simulink model "CanBusRagnarPacketLoss"  (R2021b)
settings: Solver=VariableStepAuto  StartTime=0.0  StopTime=6  RelTol=1e-3
values from neighbouring files (symbols this model uses):
  sys_mimo = ss(A,B,C,0)    [SS_MIMO.m]
libraries: truetime x6, simulink_extras x2, dspsrcs4 x1
settings Model: Creator=mozzr  LastModifiedBy=mozzr
settings SolverCC: AlgebraicLoopSolver=TrustRegion

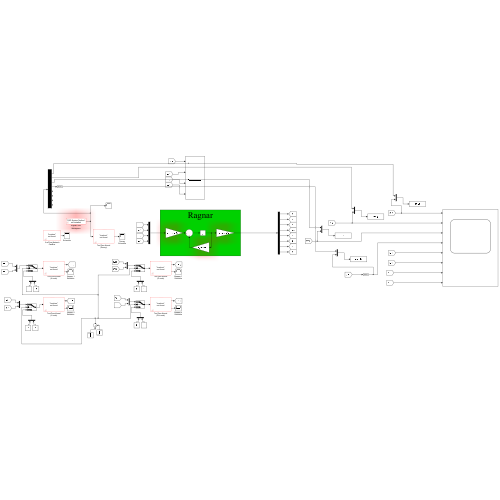
[thumbnail: Simulink's stored preview of the top-level diagram]
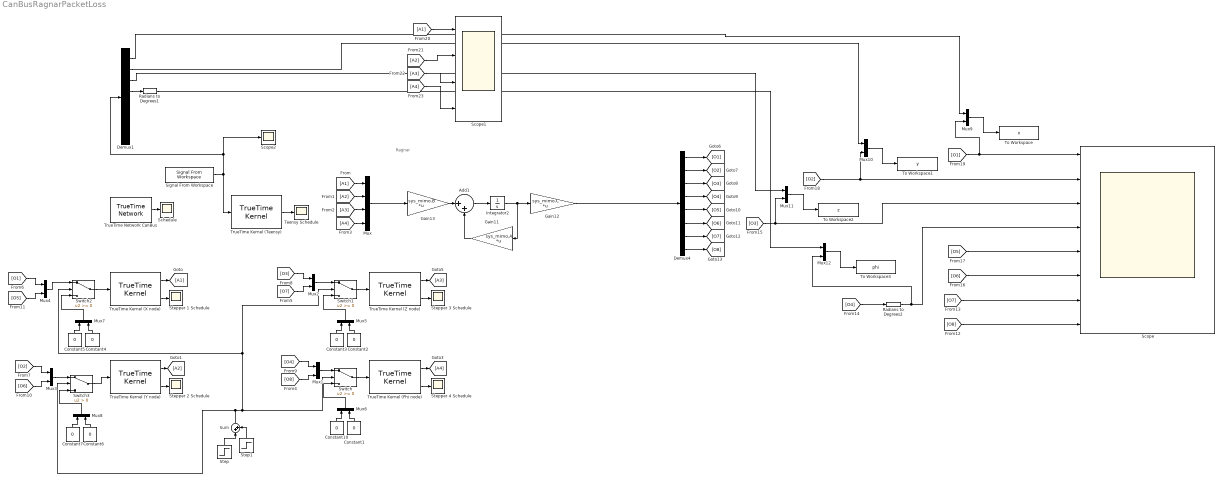
== system CanBusRagnarPacketLoss ==
  note: Ragnar
  Add1 : Sum  Inputs=|++
  Constant{1..7,10} (8 alike) : Constant  Value=0
  Demux1 : Demux  Outputs=8
  Demux4 : Demux  Outputs=8
  Gain11 : Gain  Gain=sys_mimo.A  Multiplication=Matrix(K*u)
  Gain12 : Gain  Gain=sys_mimo.C  Multiplication=Matrix(K*u)
  Gain13 : Gain  Gain=sys_mimo.B  Multiplication=Matrix(K*u)
  Integrator2 : Integrator  InitialCondition=[0 0.5 -0.4 deg2rad(90) 0 0 0 0]
  Mux : Mux
  Mux{1..12} (12 alike) : Mux  Inputs=2
  Radians to Degrees1 : simulink_extras/Transformations/Radians to Degrees
  Radians to Degrees2 : simulink_extras/Transformations/Radians to Degrees
  Schedule : Scope
  Scope : Scope  NumInputPorts=8
  Scope1 : Scope  NumInputPorts=4
  Scope2 : Scope
  Signal From Workspace : dspsrcs4/Signal From Workspace  X=ref  Ts=2  nsamps=1  OutputAfterFinalValue=Setting to zero  ignoreOrWarnInputAndFrameLengths=off  OutputFrames=off
  Step : Step  Time=1.9  Before=1  After=-1  SampleTime=0
  Step1 : Step  Time=2.15  After=2  SampleTime=0
  Stepper 1 Schedule : Scope
  Stepper 2 Schedule : Scope
  Stepper 3 Schedule : Scope
  Stepper 4 Schedule : Scope
  Sum : Sum  Inputs=|++
  Switch : Switch
  Switch1 : Switch
  Switch2 : Switch
  Switch3 : Switch  Criteria=u2 > Threshold
  Teensy Schedule : Scope
  To Workspace : ToWorkspace  VariableName=x  SaveFormat=Timeseries  SampleTime=-1
  To Workspace1 : ToWorkspace  VariableName=y  SaveFormat=Timeseries  SampleTime=-1
  To Workspace2 : ToWorkspace  VariableName=z  SaveFormat=Timeseries  SampleTime=-1
  To Workspace3 : ToWorkspace  VariableName=phi  SaveFormat=Timeseries  SampleTime=-1
  TrueTime Kernel (Phi node) : truetime/TrueTime Kernel  sfun=nodePhi_init  args=[]  ninputsoutputs=[2 1]  ntriggers=0  trigtype=falling  nwnodenbr=[1 5]  clockoffsetdrift=[0 0]  schedoutput=on  battery=off  poweroutput=off  label=1: 5
  TrueTime Kernel (Teensy) : truetime/TrueTime Kernel  sfun=Teensy_init  args=[]  ninputsoutputs=[8 0]  ntriggers=0  trigtype=falling  nwnodenbr=[1 1]  clockoffsetdrift=[0 0]  schedoutput=on  battery=off  poweroutput=off  label=1: 1
  TrueTime Kernel (X node) : truetime/TrueTime Kernel  sfun=nodeX_init  args=[]  ninputsoutputs=[2 1]  ntriggers=0  trigtype=falling  nwnodenbr=[1 2]  clockoffsetdrift=[0 0]  schedoutput=on  battery=off  poweroutput=off  label=1: 2
  TrueTime Kernel (Y node) : truetime/TrueTime Kernel  sfun=nodeY_init  args=[]  ninputsoutputs=[2 1]  ntriggers=0  trigtype=falling  nwnodenbr=[1 3]  clockoffsetdrift=[0 0]  schedoutput=on  battery=off  poweroutput=off  label=1: 3
  TrueTime Kernel (Z node) : truetime/TrueTime Kernel  sfun=nodeZ_init  args=[]  ninputsoutputs=[2 1]  ntriggers=0  trigtype=falling  nwnodenbr=[1 4]  clockoffsetdrift=[0 0]  schedoutput=on  battery=off  poweroutput=off  label=1: 4
  TrueTime Network CanBus : truetime/TrueTime Network  nwtype=CSMA/AMP (CAN)  nwnbr=1  nnodes=5  rate=10000000  minsize=512  lossprob=0  seed=0  bandwidths=[0.5 0.5]  slotsize=512  schedule=[1 1 2]  memsize=80000  buftype=Common buffer  overflow=Retransmit  dynSchedule=0  miniSlotSize=0  NIT=0  QSortMode=FIFO  sync=0  irtSchedule=0  nrtLength=0  nodeGraph=0  scheduleoutput=on
  wires:
  TrueTime Kernel (Y node)/2 -> Stepper 2 Schedule/1
  TrueTime Kernel (X node)/2 -> Stepper 1 Schedule/1
  TrueTime Kernel (Phi node)/2 -> Stepper 4 Schedule/1
  TrueTime Kernel (Z node)/2 -> Stepper 3 Schedule/1
  TrueTime Kernel (Teensy)/1 -> Teensy Schedule/1
  TrueTime Network CanBus/1 -> Schedule/1
  TrueTime Kernel (X node)/1 -> [A1]
  [A1] -> Mux/1
  TrueTime Kernel (Y node)/1 -> [A2]
  TrueTime Kernel (Phi node)/1 -> [A4]
  TrueTime Kernel (Z node)/1 -> [A3]
  [A2] -> Mux/2
  [A3] -> Mux/3
  [A4] -> Mux/4
  Demux4/1 -> [O1]
  Demux4/2 -> [O2]
  Demux4/3 -> [O3]
  Demux4/4 -> [O4]
  Demux4/5 -> [O5]
  Demux4/6 -> [O6]
  Demux4/7 -> [O7]
  Demux4/8 -> [O8]
  [O4] -> Mux1/1
  [O8] -> Mux1/2
  [O3] -> Mux2/1
  [O7] -> Mux2/2
  [O2] -> Mux3/1
  [O6] -> Mux3/2
  [O1] -> Mux4/1
  [O5] -> Mux4/2
  Gain11/1 -> Add1/2
  Gain13/1 -> Add1/1
  Add1/1 -> Integrator2/1
  Mux/1 -> Gain13/1
  Integrator2/1 -> Gain11/1, Gain12/1
  [O8] -> Scope/8
  [O7] -> Scope/7
  [O3] -> Scope/3, Mux11/2
  [O5] -> Scope/5
  [O6] -> Scope/6
  [O2] -> Mux10/2, Scope/2
  [O1] -> Mux9/2, Scope/1
  [A1] -> Scope1/1
  [A2] -> Scope1/2
  [A3] -> Scope1/3
  [A4] -> Scope1/4
  Step/1 -> Sum/1
  Step1/1 -> Sum/2
  Gain12/1 -> Demux4/1
  Mux1/1 -> Switch/1
  Sum/1 -> Switch2/2, Switch1/2, Switch/2, Switch3/2
  Mux6/1 -> Switch/3
  Constant10/1 -> Mux6/1
  Constant1/1 -> Mux6/2
  Switch/1 -> TrueTime Kernel (Phi node)/1
  Mux5/1 -> Switch1/3
  Constant3/1 -> Mux5/1
  Constant2/1 -> Mux5/2
  Mux2/1 -> Switch1/1
  Switch1/1 -> TrueTime Kernel (Z node)/1
  Mux7/1 -> Switch2/3
  Constant5/1 -> Mux7/1
  Constant4/1 -> Mux7/2
  Mux4/1 -> Switch2/1
  Switch2/1 -> TrueTime Kernel (X node)/1
  Mux8/1 -> Switch3/3
  Constant7/1 -> Mux8/1
  Constant6/1 -> Mux8/2
  Mux3/1 -> Switch3/1
  Switch3/1 -> TrueTime Kernel (Y node)/1
  Signal From Workspace/1 -> TrueTime Kernel (Teensy)/1, Scope2/1, Demux1/1
  Demux1/3 -> Mux11/1
  Demux1/1 -> Mux9/1
  Radians to Degrees1/1 -> Mux12/1
  Demux1/4 -> Radians to Degrees1/1
  Demux1/2 -> Mux10/1
  Mux9/1 -> To Workspace/1
  Mux10/1 -> To Workspace1/1
  Mux11/1 -> To Workspace2/1
  Mux12/1 -> To Workspace3/1
  [O4] -> Radians to Degrees2/1
  Radians to Degrees2/1 -> Mux12/2, Scope/4
